simulink model "vienna_practice"  (Simulink 7.6)
settings: Solver=ode45  StartTime=0.0  StopTime=40e-3  RelTol=1e-3
libraries: powerlib_extras x1, powerlib x1
settings Model: Creator=huanglei  LastModifiedBy=huanglei

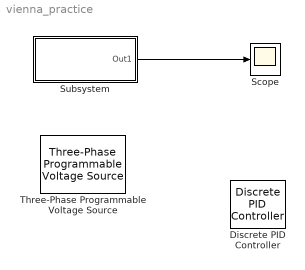
== system vienna_practice ==
  Discrete PID Controller : powerlib_extras/Discrete  Control Blocks/Discrete PID Controller  DialogController=POWERSYS.PowerSysDialog  SystemSampleTime=-1  Kp=1  Ki=1  Kd=1  TcD=1  Par_Limits=[100 -100]  Init=0  Ts=0.5
  Scope : Scope
      settings: SaveName=sine  DataFormat=Array
  Subsystem : Subsystem
  Three-Phase Programmable Voltage Source : powerlib/Electrical Sources/Three-Phase Programmable Voltage Source  DialogController=POWERSYS.PowerSysDialog  SystemSampleTime=-1  PositiveSequence="[100  0 60]"  VariationEntity=None  VariationType=Step  VariationStep=0.5  VariationRate=10  VariationMagnitude=0.3  VariationFrequency=2  VariationTiming=[1 2]  VariationPhaseA=off  Amplitudes=[1 0.8 1.2 1.0]  TimeValues=[0 0.1 0.15 0.2]  HarmonicGeneration=off  HarmonicA=[3 0.2 -25 0]  HarmonicB=[2 0.15 35 2]  Timing="[0.05  3]"
  wires:
  Subsystem/1(Out1) -> Scope/1

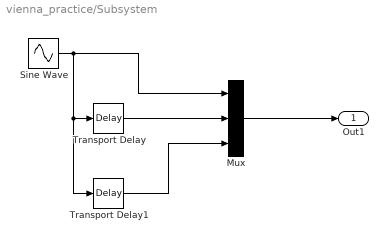
== system vienna_practice/Subsystem ==
  Mux : Mux  Inputs=3
  Sine Wave : Sin  Amplitude=220  Frequency=314  SampleTime=0
  Transport Delay : TransportDelay  DelayTime=0.02/3
  Transport Delay1 : TransportDelay  DelayTime=0.04/3
  Out1 : Outport
  wires:
  Sine Wave/1 -> Mux/1, Transport Delay/1, Transport Delay1/1
  Transport Delay/1 -> Mux/2
  Transport Delay1/1 -> Mux/3
  Mux/1 -> Out1/1
